simulink model "rpoco16"  (R2013a)
settings: Solver=VariableStepDiscrete  SolverMode=SingleTasking  StartTime=0.0  StopTime=10.0  RelTol=1e-3
libraries: xbsIndex_r4 x7152, casper_library_misc x156, casper_library_multipliers x68, casper_library_sources x8, xps_library x5, casper_library_delays x1
(part 2 of 84)

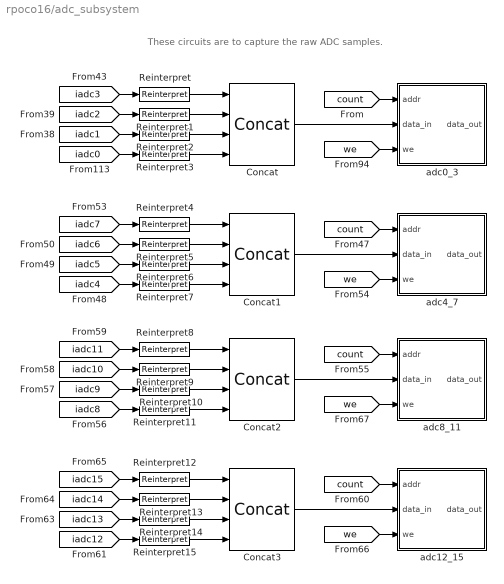
== system rpoco16/adc_subsystem ==
  note: These circuits are to capture the raw ADC samples.
  Concat{,1..3} (4 alike) : xbsIndex_r4/Concat  num_inputs=4  dbl_ovrd=off  block_type=concat
  Reinterpret{,1..15} (16 alike) : xbsIndex_r4/Reinterpret  force_arith_type=on  arith_type=Unsigned  force_bin_pt=on  bin_pt=0  block_type=reinterpret
      settings: infoedit="Changes signal type without altering the binary representation.   You can changed the signal between signed and unsigned, and relocate the binary point.<br><br>Hardware notes: In hardware this block costs nothing.<br><br>Example:  Suppose the input is 6 bits wide, signed, with 2 fractional bits, and the output is forced to unsigned with 0 fractional bits.  Then an input of -2.0 (1110.00 in binary 2's complement) becomes an output of 56 (111000 in binary)."
  adc0_3 : Subsystem  Tag=xps:bram  AncestorBlock=xps_library/Shared BRAM  mask{arith_type=Unsigned, addr_width=11, data_width=32, reg_prim_output=off, reg_core_output=off, optimization=Minimum_Area, data_bin_pt=0, init_vals=[1:2^10-1], sample_rate=1}
      mask prompts: arith_type "Output Data Type"; addr_width "Address width"; data_width "Data Width"; reg_prim_output "Register Primitive Output"; reg_core_output "Register Core Output"; data_bin_pt "Data Binary Point"; init_vals "Initial values (simulation only)"; sample_rate "Sample rate"
      mask init:
      | shared_bram_mask;
      mask TypeOptions arith_type: Unsigned | Signed  (2's comp)
      mask TypeOptions data_width: 8 | 16 | 32 | 64 | 128
      mask TypeOptions optimization: Minimum_Area | Low_Power
  adc12_15 : Subsystem  Tag=xps:bram  AncestorBlock=xps_library/Shared BRAM  mask{arith_type=Unsigned, addr_width=11, data_width=32, reg_prim_output=off, reg_core_output=off, optimization=Minimum_Area, data_bin_pt=0, init_vals=[1:2^10-1], sample_rate=1}
      mask prompts: arith_type "Output Data Type"; addr_width "Address width"; data_width "Data Width"; reg_prim_output "Register Primitive Output"; reg_core_output "Register Core Output"; data_bin_pt "Data Binary Point"; init_vals "Initial values (simulation only)"; sample_rate "Sample rate"
      mask init:
      | shared_bram_mask;
      mask TypeOptions arith_type: Unsigned | Signed  (2's comp)
      mask TypeOptions data_width: 8 | 16 | 32 | 64 | 128
      mask TypeOptions optimization: Minimum_Area | Low_Power
  adc4_7 : Subsystem  Tag=xps:bram  AncestorBlock=xps_library/Shared BRAM  mask{arith_type=Unsigned, addr_width=11, data_width=32, reg_prim_output=off, reg_core_output=off, optimization=Minimum_Area, data_bin_pt=0, init_vals=[1:2^10-1], sample_rate=1}
      mask prompts: arith_type "Output Data Type"; addr_width "Address width"; data_width "Data Width"; reg_prim_output "Register Primitive Output"; reg_core_output "Register Core Output"; data_bin_pt "Data Binary Point"; init_vals "Initial values (simulation only)"; sample_rate "Sample rate"
      mask init:
      | shared_bram_mask;
      mask TypeOptions arith_type: Unsigned | Signed  (2's comp)
      mask TypeOptions data_width: 8 | 16 | 32 | 64 | 128
      mask TypeOptions optimization: Minimum_Area | Low_Power
  adc8_11 : Subsystem  Tag=xps:bram  AncestorBlock=xps_library/Shared BRAM  mask{arith_type=Unsigned, addr_width=11, data_width=32, reg_prim_output=off, reg_core_output=off, optimization=Minimum_Area, data_bin_pt=0, init_vals=[1:2^10-1], sample_rate=1}
      mask prompts: arith_type "Output Data Type"; addr_width "Address width"; data_width "Data Width"; reg_prim_output "Register Primitive Output"; reg_core_output "Register Core Output"; data_bin_pt "Data Binary Point"; init_vals "Initial values (simulation only)"; sample_rate "Sample rate"
      mask init:
      | shared_bram_mask;
      mask TypeOptions arith_type: Unsigned | Signed  (2's comp)
      mask TypeOptions data_width: 8 | 16 | 32 | 64 | 128
      mask TypeOptions optimization: Minimum_Area | Low_Power
  wires:
  [count] -> adc4_7/1(addr)
  [we] -> adc4_7/3(we)
  Concat1/1 -> adc4_7/2(data_in)
  Reinterpret4/1 -> Concat1/1
  Reinterpret5/1 -> Concat1/2
  Reinterpret6/1 -> Concat1/3
  Reinterpret7/1 -> Concat1/4
  [iadc7] -> Reinterpret4/1
  [iadc6] -> Reinterpret5/1
  [iadc5] -> Reinterpret6/1
  [iadc4] -> Reinterpret7/1
  Reinterpret13/1 -> Concat3/2
  Reinterpret14/1 -> Concat3/3
  Reinterpret15/1 -> Concat3/4
  [iadc15] -> Reinterpret12/1
  [iadc14] -> Reinterpret13/1
  [iadc13] -> Reinterpret14/1
  [iadc12] -> Reinterpret15/1
  Reinterpret8/1 -> Concat2/1
  Reinterpret9/1 -> Concat2/2
  Reinterpret10/1 -> Concat2/3
  Reinterpret11/1 -> Concat2/4
  [iadc11] -> Reinterpret8/1
  [iadc10] -> Reinterpret9/1
  [iadc9] -> Reinterpret10/1
  [iadc8] -> Reinterpret11/1
  [count] -> adc12_15/1(addr)
  [we] -> adc12_15/3(we)
  Reinterpret12/1 -> Concat3/1
  Concat3/1 -> adc12_15/2(data_in)
  [count] -> adc8_11/1(addr)
  Concat2/1 -> adc8_11/2(data_in)
  [we] -> adc8_11/3(we)
  Reinterpret2/1 -> Concat/3
  Reinterpret1/1 -> Concat/2
  [iadc3] -> Reinterpret/1
  Reinterpret/1 -> Concat/1
  [iadc1] -> Reinterpret2/1
  Reinterpret3/1 -> Concat/4
  Concat/1 -> adc0_3/2(data_in)
  [count] -> adc0_3/1(addr)
  [we] -> adc0_3/3(we)
  [iadc0] -> Reinterpret3/1
  [iadc2] -> Reinterpret1/1

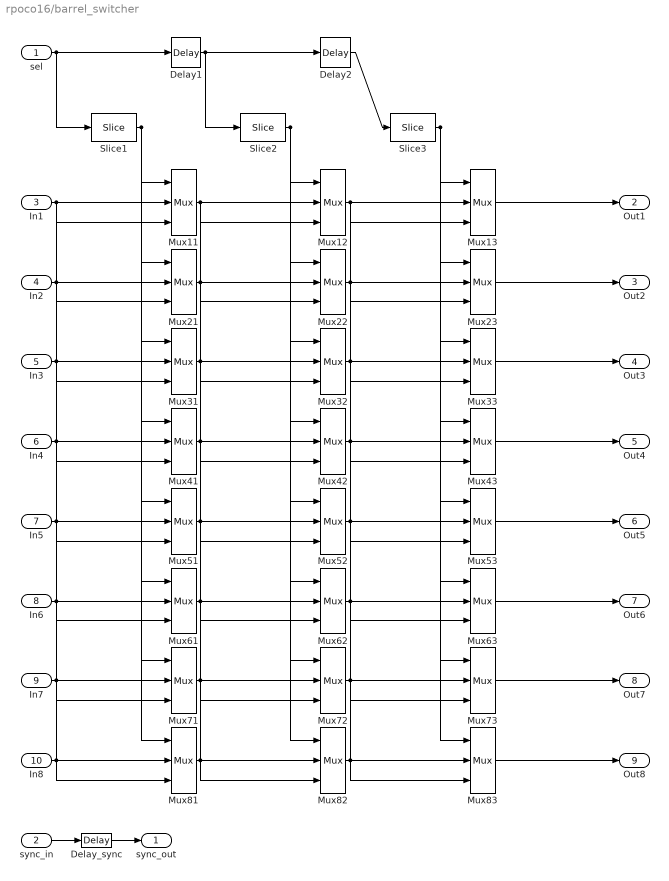
== system rpoco16/barrel_switcher ==
  sel : Inport
  sync_in : Inport  Port=2
  In1 : Inport  Port=3
  In2 : Inport  Port=4
  In3 : Inport  Port=5
  In4 : Inport  Port=6
  In5 : Inport  Port=7
  In6 : Inport  Port=8
  In7 : Inport  Port=9
  In8 : Inport  Port=10
  Delay1 : xbsIndex_r4/Delay  rst=off  infoeditControl=Selection of Reset will increase slice count due to use of real FFs and instead of SRLs  en=off  latency=1  dbl_ovrd=off  reg_retiming=on  block_type=delay
  Delay2 : xbsIndex_r4/Delay  rst=off  infoeditControl=Selection of Reset will increase slice count due to use of real FFs and instead of SRLs  en=off  latency=1  dbl_ovrd=off  reg_retiming=on  block_type=delay
  Delay_sync : xbsIndex_r4/Delay  rst=off  infoeditControl=Selection of Reset will increase slice count due to use of real FFs and instead of SRLs  en=off  latency=3  dbl_ovrd=off  reg_retiming=on  block_type=delay
  Mux{11..13,21..23,31..33,41..43,51..53,61..63,71..73,81..83} (24 alike) : xbsIndex_r4/Mux  inputs=2  en=off  latency=1  precision=Full  arith_type=Unsigned  n_bits=16  bin_pt=14  quantization=Truncate  overflow=Wrap  dbl_ovrd=off  block_type=mux
  Slice1 : xbsIndex_r4/Slice  nbits=1  boolean_output=off  mode=Upper Bit Location + Width  bit1=-0  base1=MSB of Input  bit0=0  base0=LSB of Input  dbl_ovrd=off  block_type=slice
  Slice2 : xbsIndex_r4/Slice  nbits=1  boolean_output=off  mode=Upper Bit Location + Width  bit1=-1  base1=MSB of Input  bit0=0  base0=LSB of Input  dbl_ovrd=off  block_type=slice
  Slice3 : xbsIndex_r4/Slice  nbits=1  boolean_output=off  mode=Upper Bit Location + Width  bit1=-2  base1=MSB of Input  bit0=0  base0=LSB of Input  dbl_ovrd=off  block_type=slice
  sync_out : Outport
  Out1 : Outport  Port=2
  Out2 : Outport  Port=3
  Out3 : Outport  Port=4
  Out4 : Outport  Port=5
  Out5 : Outport  Port=6
  Out6 : Outport  Port=7
  Out7 : Outport  Port=8
  Out8 : Outport  Port=9
  wires:
  sync_in/1 -> Delay_sync/1
  Delay_sync/1 -> sync_out/1
  sel/1 -> Slice1/1, Delay1/1
  Delay1/1 -> Delay2/1, Slice2/1
  Delay2/1 -> Slice3/1
  Slice1/1 -> Mux11/1, Mux21/1, Mux31/1, Mux41/1, Mux51/1, Mux61/1, Mux71/1, Mux81/1
  Slice2/1 -> Mux12/1, Mux22/1, Mux32/1, Mux42/1, Mux52/1, Mux62/1, Mux72/1, Mux82/1
  Slice3/1 -> Mux13/1, Mux23/1, Mux33/1, Mux43/1, Mux53/1, Mux63/1, Mux73/1, Mux83/1
  In1/1 -> Mux11/2, Mux51/3
  Mux13/1 -> Out1/1
  In2/1 -> Mux21/2, Mux61/3
  Mux23/1 -> Out2/1
  In3/1 -> Mux31/2, Mux71/3
  Mux33/1 -> Out3/1
  In4/1 -> Mux41/2, Mux81/3
  Mux43/1 -> Out4/1
  In5/1 -> Mux51/2, Mux11/3
  Mux53/1 -> Out5/1
  In6/1 -> Mux61/2, Mux21/3
  Mux63/1 -> Out6/1
  In7/1 -> Mux71/2, Mux31/3
  Mux73/1 -> Out7/1
  In8/1 -> Mux81/2, Mux41/3
  Mux83/1 -> Out8/1
  Mux11/1 -> Mux12/2, Mux72/3
  Mux12/1 -> Mux13/2, Mux83/3
  Mux21/1 -> Mux22/2, Mux82/3
  Mux22/1 -> Mux23/2, Mux13/3
  Mux31/1 -> Mux32/2, Mux12/3
  Mux32/1 -> Mux33/2, Mux23/3
  Mux41/1 -> Mux42/2, Mux22/3
  Mux42/1 -> Mux43/2, Mux33/3
  Mux51/1 -> Mux52/2, Mux32/3
  Mux52/1 -> Mux53/2, Mux43/3
  Mux61/1 -> Mux62/2, Mux42/3
  Mux62/1 -> Mux63/2, Mux53/3
  Mux71/1 -> Mux72/2, Mux52/3
  Mux72/1 -> Mux73/2, Mux63/3
  Mux81/1 -> Mux82/2, Mux62/3
  Mux82/1 -> Mux83/2, Mux73/3

== system rpoco16/ctrl_sw ==
  sim_1 : Inport
  io_delay : xbsIndex_r4/Delay  rst=off  infoeditControl=Selection of Reset will increase slice count due to use of real FFs and instead of SRLs  en=off  latency=0  dbl_ovrd=off  reg_retiming=on  block_type=delay
  reint1 : xbsIndex_r4/Reinterpret  force_arith_type=on  arith_type=Unsigned  force_bin_pt=on  bin_pt=0  block_type=reinterpret
  rpoco16_ctrl_sw_user_data_out : xbsIndex_r4/Gateway In  gui_display_data_type=Fixed-point  arith_type=Unsigned  n_bits=32  bin_pt=0  preci_type=Single  exp_width=8  frac_width=24  quantization="Round  (unbiased: +/- Inf)"  overflow=Saturate  period=1  dbl_ovrd=off  timing_constraint=None  locs_specified=off  LOCs={}  UseAsADC=off  ADCChannel='1'  inherit_from_input=off  hdl_port=on  block_type=gatewayin
  slice_reg : xbsIndex_r4/Slice  nbits=32  boolean_output=off  mode=Lower Bit Location + Width  bit1=0  base1=MSB of Input  bit0=0  base0=LSB of Input  dbl_ovrd=off  block_type=slice
  in_reg : Outport
  wires:
  rpoco16_ctrl_sw_user_data_out/1 -> io_delay/1
  sim_1/1 -> rpoco16_ctrl_sw_user_data_out/1
  io_delay/1 -> slice_reg/1
  slice_reg/1 -> reint1/1
  reint1/1 -> in_reg/1

== system rpoco16/delay ==
  note: Delay data is a 32 bit input, and delayi is a
      | 4 bit output. Max delay is 16 clocks.
  BitBasher : xbsIndex_r4/BitBasher  bitexpr=|  display_expr=off  sr_1=1  arith_type1=Unsigned  bin_pt1=0  sr_2=2  arith_type2=Unsigned  bin_pt2=0  sr_3=3  arith_type3=Unsigned  bin_pt3=0  sr_4=4  arith_type4=Unsigned  bin_pt4=0  dbl_ovrd=off  block_type=bitbasher
      | <html><head><meta name="qrichtext" content="1" /><style type="text/css">
      | p, li { white-space: pre-wrap; }
      | </style></head><body style=" font-family:'MS Shell Dlg 2'; font-size:8.25pt; font-weight:400; font-style:normal;">
      | <p style=" margin-top:12px; margin-bottom:12px; margin-left:0px; margin-right:0px; -qt-block-indent:0; text-indent:0px; font-family:'MS Shell Dlg'; font-size:8pt;">delay0={delay[3:0]}<br />delay1={delay[7:4]}<br />delay2={delay[11:8]}<br />delay3={delay[15:12]}</p></body></html>
      settings: block_version=10.1.3
  BitBasher1 : xbsIndex_r4/BitBasher  bitexpr=|  display_expr=off  sr_1=1  arith_type1=Unsigned  bin_pt1=0  sr_2=2  arith_type2=Unsigned  bin_pt2=0  sr_3=3  arith_type3=Unsigned  bin_pt3=0  sr_4=4  arith_type4=Unsigned  bin_pt4=0  dbl_ovrd=off  block_type=bitbasher
      | <html><head><meta name="qrichtext" content="1" /><style type="text/css">
      | p, li { white-space: pre-wrap; }
      | </style></head><body style=" font-family:'MS Shell Dlg 2'; font-size:8.25pt; font-weight:400; font-style:normal;">
      | <p style=" margin-top:12px; margin-bottom:12px; margin-left:0px; margin-right:0px; -qt-block-indent:0; text-indent:0px; font-family:'MS Shell Dlg'; font-size:8pt;">delay4={delay[19:16]}<br />delay5={delay[23:20]}<br />delay6={delay[27:24]}<br />delay7={delay[31:28]}</p></body></html>
      settings: block_version=10.1.3
  Constant : Constant
  delay_data : Subsystem  Tag=xps:sw_reg  AncestorBlock=xps_library/software register  mask(swreg){mode=one value, io_dir=From Processor, io_delay=0, sample_period=1, names=reg, bitwidths=32, arith_types=0, bin_pts=0, sim_port=on, show_format=off}
      mask prompts: io_dir "I/O direction"; io_delay "I/O delay"; sample_period "Sample period"; names "Name:"; bitwidths "Bitwidth:"; arith_types "Type (ufix=0, fix=1, bool=2):"; bin_pts "Binary pt:"; sim_port "Provide sim input/output?"; show_format "Print format string?"
      mask init:
      | swreg_init(gcb)
      settings: AttributesFormatString=1input
      mask TypeOptions mode: one value | fields of equal size | fields of arbitrary size
      mask Callback mode: swreg_cb(gcb);
      mask TypeOptions io_dir: To Processor | From Processor
      mask Callback io_dir:
      | mask_enables = get_param(gcb, 'MaskEnables');
      | mask_names = get_param(gcb, 'MaskNames');
      | if strcmp(get_param(gcb, 'io_dir'), 'To Processor'),
      |     mask_enables{ismember(mask_names, 'sample_period')} = 'off';
      | else
      |     mask_enables{ismember(mask_names, 'sample_period')} = 'on';
      | end
      | set_param(gcb, 'MaskEnables', mask_enables);
      mask Callback bitwidths: swreg_maskcheck(gcb);
      mask Callback arith_types: [numios, ~, ~, ~, current_types] = swreg_maskcheck(gcb);
      mask Callback bin_pts: swreg_maskcheck(gcb);
  tag scope: delay0=global, delay10=global, delay11=global, delay12=global, delay13=global, delay14=global, delay15=global, delay1=global, delay2=global, delay3=global, delay4=global, delay5=global, delay6=global, delay7=global, delay8=global, delay9=global
  wires:
  delay_data/1(in_reg) -> BitBasher1/1, BitBasher/1
  Constant/1 -> delay_data/1(sim_1)
  BitBasher/1 -> [delay1], [delay0]
  BitBasher/2 -> [delay3], [delay2]
  BitBasher/3 -> [delay5], [delay4]
  BitBasher/4 -> [delay7], [delay6]
  BitBasher1/1 -> [delay9], [delay8]
  BitBasher1/2 -> [delay11], [delay10]
  BitBasher1/3 -> [delay13], [delay12]
  BitBasher1/4 -> [delay15], [delay14]

== system rpoco16/edge ==
  in : Inport
  Delay : xbsIndex_r4/Delay  rst=off  infoeditControl=Selection of Reset will increase slice count due to use of real FFs and instead of SRLs  en=off  latency=1  dbl_ovrd=off  reg_retiming=off  block_type=delay
      settings: xl_area=[0, 0, 0, 0, 0, 0, 0]
  Inverter : xbsIndex_r4/Inverter  en=off  latency=0  dbl_ovrd=off  block_type=inv
      settings: xl_area=[0, 0, 0, 0, 0, 0, 0]
  edge_op : xbsIndex_r4/Logical  logical_function=XNOR  inputs=2  en=off  latency=0  precision=Full  arith_type=Unsigned  n_bits=8  bin_pt=2  align_bp=on  dbl_ovrd=off  block_type=logical
      settings: xl_area=[0, 0, 0, 0, 0, 0, 0]
  out : Outport
  wires:
  Inverter/1 -> edge_op/1
  edge_op/1 -> out/1
  in/1 -> Inverter/1, Delay/1
  Delay/1 -> edge_op/2

== system rpoco16/eq_coeff ==
  sim_1 : Inport
  io_delay : xbsIndex_r4/Delay  rst=off  infoeditControl=Selection of Reset will increase slice count due to use of real FFs and instead of SRLs  en=off  latency=0  dbl_ovrd=off  reg_retiming=on  block_type=delay
  reint1 : xbsIndex_r4/Reinterpret  force_arith_type=on  arith_type=Unsigned  force_bin_pt=on  bin_pt=0  block_type=reinterpret
  rpoco16_eq_coeff_user_data_out : xbsIndex_r4/Gateway In  gui_display_data_type=Fixed-point  arith_type=Unsigned  n_bits=32  bin_pt=0  preci_type=Single  exp_width=8  frac_width=24  quantization="Round  (unbiased: +/- Inf)"  overflow=Saturate  period=1  dbl_ovrd=off  timing_constraint=None  locs_specified=off  LOCs={}  UseAsADC=off  ADCChannel='1'  inherit_from_input=off  hdl_port=on  block_type=gatewayin
  slice_reg : xbsIndex_r4/Slice  nbits=32  boolean_output=off  mode=Lower Bit Location + Width  bit1=0  base1=MSB of Input  bit0=0  base0=LSB of Input  dbl_ovrd=off  block_type=slice
  in_reg : Outport
  wires:
  rpoco16_eq_coeff_user_data_out/1 -> io_delay/1
  sim_1/1 -> rpoco16_eq_coeff_user_data_out/1
  io_delay/1 -> slice_reg/1
  slice_reg/1 -> reint1/1
  reint1/1 -> in_reg/1

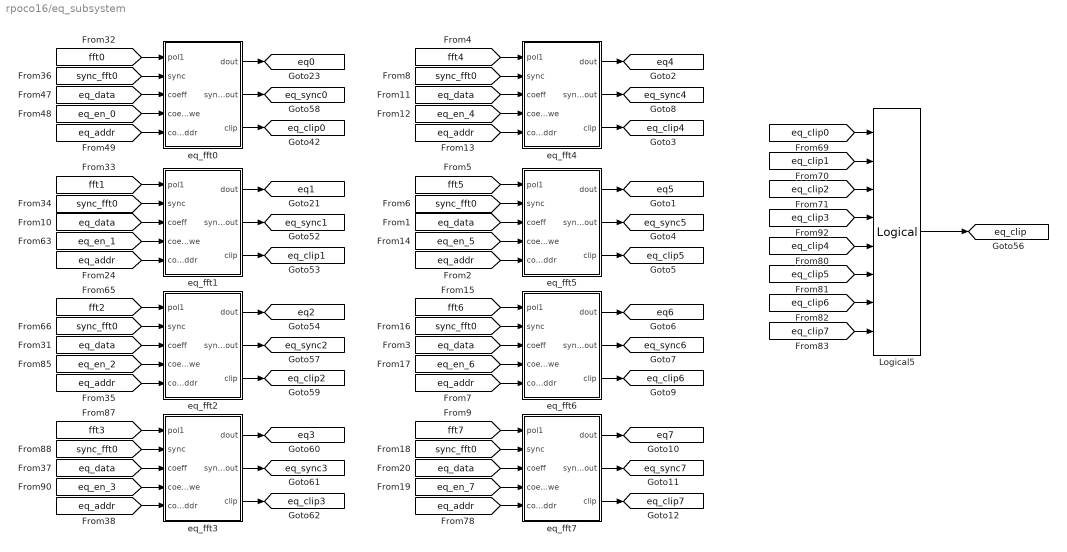
== system rpoco16/eq_subsystem ==
  Logical5 : xbsIndex_r4/Logical  logical_function=OR  inputs=8  en=off  latency=0  precision=Full  arith_type=Unsigned  n_bits=8  bin_pt=2  align_bp=on  dbl_ovrd=off  block_type=logical
      settings: xl_area=[0, 0, 0, 0, 0, 0, 0]
  eq_fft0 : Subsystem  mask{nchan=11}
      mask prompts: nchan "FFT Channels (2^?):"
  eq_fft1 : Subsystem  mask{nchan=11}
      mask prompts: nchan "FFT Channels (2^?):"
  eq_fft2 : Subsystem  mask{nchan=11}
      mask prompts: nchan "FFT Channels (2^?):"
  eq_fft3 : Subsystem  mask{nchan=11}
      mask prompts: nchan "FFT Channels (2^?):"
  eq_fft4 : Subsystem  mask{nchan=11}
      mask prompts: nchan "FFT Channels (2^?):"
  eq_fft5 : Subsystem  mask{nchan=11}
      mask prompts: nchan "FFT Channels (2^?):"
  eq_fft6 : Subsystem  mask{nchan=11}
      mask prompts: nchan "FFT Channels (2^?):"
  eq_fft7 : Subsystem  mask{nchan=11}
      mask prompts: nchan "FFT Channels (2^?):"
  tag scope: eq0=global, eq1=global, eq2=global, eq3=global, eq4=global, eq5=global, eq6=global, eq7=global, eq_clip0=global, eq_clip1=global, eq_clip2=global, eq_clip3=global, eq_clip4=global, eq_clip5=global, eq_clip6=global, eq_clip7=global, eq_clip=global, eq_sync0=global, eq_sync1=global, eq_sync2=global, eq_sync3=global, eq_sync4=global, eq_sync5=global, eq_sync6=global, eq_sync7=global
  wires:
  Logical5/1 -> [eq_clip]
  [eq_clip0] -> Logical5/1
  [eq_clip1] -> Logical5/2
  [eq_clip2] -> Logical5/3
  [eq_clip3] -> Logical5/4
  [eq_data] -> eq_fft1/3(coeff)
  eq_fft0/1(dout) -> [eq0]
  eq_fft0/2(sync_out) -> [eq_sync0]
  [fft0] -> eq_fft0/1(pol1)
  [eq_data] -> eq_fft0/3(coeff)
  [eq_en_0] -> eq_fft0/4(coeff_we)
  eq_fft0/3(clip) -> [eq_clip0]
  [sync_fft0] -> eq_fft0/2(sync)
  [eq_addr] -> eq_fft0/5(coeff_addr)
  [fft1] -> eq_fft1/1(pol1)
  [sync_fft0] -> eq_fft1/2(sync)
  [eq_en_1] -> eq_fft1/4(coeff_we)
  [eq_addr] -> eq_fft1/5(coeff_addr)
  [fft2] -> eq_fft2/1(pol1)
  [sync_fft0] -> eq_fft2/2(sync)
  [eq_data] -> eq_fft2/3(coeff)
  [eq_en_2] -> eq_fft2/4(coeff_we)
  [eq_addr] -> eq_fft2/5(coeff_addr)
  [fft3] -> eq_fft3/1(pol1)
  [sync_fft0] -> eq_fft3/2(sync)
  [eq_data] -> eq_fft3/3(coeff)
  [eq_en_3] -> eq_fft3/4(coeff_we)
  [eq_addr] -> eq_fft3/5(coeff_addr)
  eq_fft1/1(dout) -> [eq1]
  eq_fft1/2(sync_out) -> [eq_sync1]
  eq_fft1/3(clip) -> [eq_clip1]
  eq_fft2/1(dout) -> [eq2]
  eq_fft2/2(sync_out) -> [eq_sync2]
  eq_fft2/3(clip) -> [eq_clip2]
  eq_fft3/1(dout) -> [eq3]
  eq_fft3/2(sync_out) -> [eq_sync3]
  eq_fft3/3(clip) -> [eq_clip3]
  [eq_data] -> eq_fft5/3(coeff)
  eq_fft4/1(dout) -> [eq4]
  eq_fft4/2(sync_out) -> [eq_sync4]
  [fft4] -> eq_fft4/1(pol1)
  [eq_data] -> eq_fft4/3(coeff)
  [eq_en_4] -> eq_fft4/4(coeff_we)
  eq_fft4/3(clip) -> [eq_clip4]
  [sync_fft0] -> eq_fft4/2(sync)
  [eq_addr] -> eq_fft4/5(coeff_addr)
  [fft5] -> eq_fft5/1(pol1)
  [sync_fft0] -> eq_fft5/2(sync)
  [eq_en_5] -> eq_fft5/4(coeff_we)
  [eq_addr] -> eq_fft5/5(coeff_addr)
  [fft6] -> eq_fft6/1(pol1)
  [sync_fft0] -> eq_fft6/2(sync)
  [eq_data] -> eq_fft6/3(coeff)
  [eq_en_6] -> eq_fft6/4(coeff_we)
  [eq_addr] -> eq_fft6/5(coeff_addr)
  eq_fft5/1(dout) -> [eq5]
  eq_fft5/2(sync_out) -> [eq_sync5]
  eq_fft5/3(clip) -> [eq_clip5]
  eq_fft6/1(dout) -> [eq6]
  eq_fft6/2(sync_out) -> [eq_sync6]
  eq_fft6/3(clip) -> [eq_clip6]
  [fft7] -> eq_fft7/1(pol1)
  [sync_fft0] -> eq_fft7/2(sync)
  [eq_data] -> eq_fft7/3(coeff)
  [eq_en_7] -> eq_fft7/4(coeff_we)
  [eq_addr] -> eq_fft7/5(coeff_addr)
  eq_fft7/1(dout) -> [eq7]
  eq_fft7/2(sync_out) -> [eq_sync7]
  eq_fft7/3(clip) -> [eq_clip7]
  [eq_clip4] -> Logical5/5
  [eq_clip5] -> Logical5/6
  [eq_clip6] -> Logical5/7
  [eq_clip7] -> Logical5/8

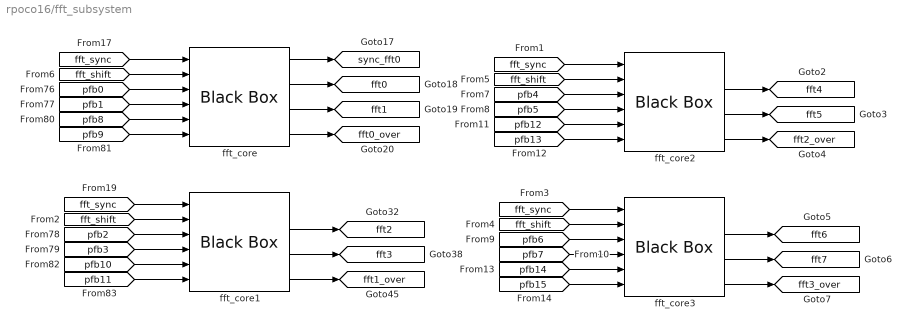
== system rpoco16/fft_subsystem ==
  fft_core{,1..3} (4 alike) : xbsIndex_r4/Black Box  init_code=fft_core_v6_config  sim_method=Inactive  verbose=off  block_type=blackbox2
  tag scope: fft0=global, fft0_over=global, fft1=global, fft1_over=global, fft2=global, fft2_over=global, fft3=global, fft3_over=global, fft4=global, fft5=global, fft6=global, fft7=global, sync_fft0=global
  wires:
  [pfb1] -> fft_core/4
  [pfb11] -> fft_core1/6
  [pfb3] -> fft_core1/4
  [pfb0] -> fft_core/3
  fft_core/4 -> [fft0_over]
  [fft_sync] -> fft_core/1
  [pfb8] -> fft_core/5
  fft_core1/3 -> [fft3]
  fft_core/2 -> [fft0]
  [pfb2] -> fft_core1/3
  [fft_sync] -> fft_core1/1
  [pfb9] -> fft_core/6
  fft_core1/4 -> [fft1_over]
  [fft_shift] -> fft_core/2
  fft_core1/2 -> [fft2]
  [fft_shift] -> fft_core1/2
  fft_core/3 -> [fft1]
  [pfb10] -> fft_core1/5
  fft_core/1 -> [sync_fft0]
  [pfb5] -> fft_core2/4
  [pfb15] -> fft_core3/6
  [pfb7] -> fft_core3/4
  [pfb4] -> fft_core2/3
  fft_core2/4 -> [fft2_over]
  [fft_sync] -> fft_core2/1
  [pfb12] -> fft_core2/5
  fft_core3/3 -> [fft7]
  fft_core2/2 -> [fft4]
  [pfb6] -> fft_core3/3
  [fft_sync] -> fft_core3/1
  [pfb13] -> fft_core2/6
  fft_core3/4 -> [fft3_over]
  [fft_shift] -> fft_core2/2
  fft_core3/2 -> [fft6]
  [fft_shift] -> fft_core3/2
  fft_core2/3 -> [fft5]
  [pfb14] -> fft_core3/5

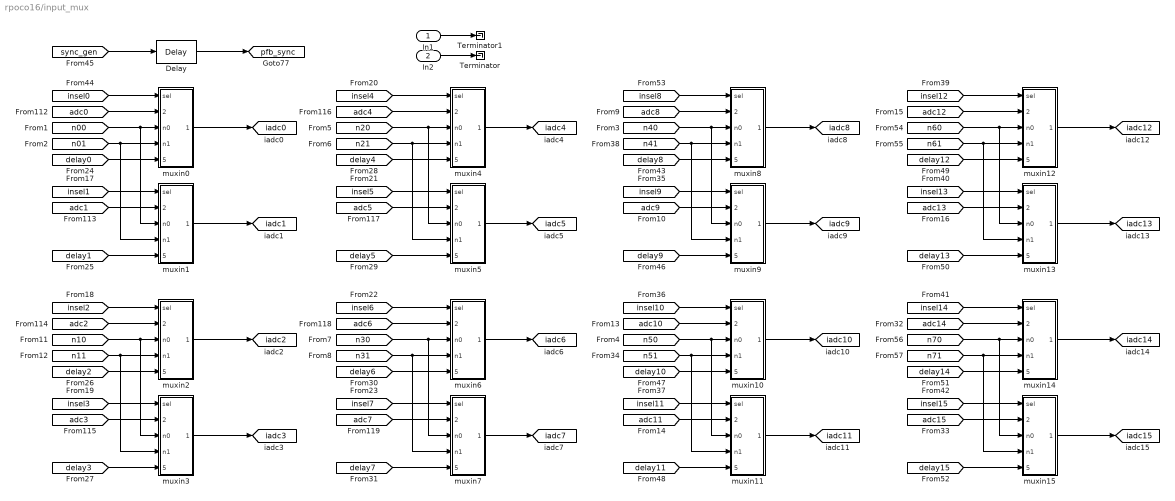
== system rpoco16/input_mux ==
  In1 : Inport
  In2 : Inport  Port=2
  Delay : xbsIndex_r4/Delay  rst=off  infoeditControl=Selection of Reset will increase slice count due to use of real FFs and instead of SRLs  en=off  latency=2  dbl_ovrd=off  reg_retiming=off  block_type=delay
  Terminator : Terminator
  Terminator1 : Terminator
  muxin0 : Subsystem
  muxin1 : Subsystem
  muxin10 : Subsystem
  muxin11 : Subsystem
  muxin12 : Subsystem
  muxin13 : Subsystem
  muxin14 : Subsystem
  muxin15 : Subsystem
  muxin2 : Subsystem
  muxin3 : Subsystem
  muxin4 : Subsystem
  muxin5 : Subsystem
  muxin6 : Subsystem
  muxin7 : Subsystem
  muxin8 : Subsystem
  muxin9 : Subsystem
  tag scope: iadc0=global, iadc10=global, iadc11=global, iadc12=global, iadc13=global, iadc14=global, iadc15=global, iadc1=global, iadc2=global, iadc3=global, iadc4=global, iadc5=global, iadc6=global, iadc7=global, iadc8=global, iadc9=global, pfb_sync=global
  wires:
  [insel0] -> muxin0/1(sel)
  [adc0] -> muxin0/2(adc)
  [n00] -> muxin0/3(n0), muxin1/3(n0)
  [n01] -> muxin0/4(n1), muxin1/4(n1)
  [delay0] -> muxin0/5(delay)
  [insel1] -> muxin1/1(sel)
  [adc1] -> muxin1/2(adc)
  [delay1] -> muxin1/5(delay)
  [insel2] -> muxin2/1(sel)
  [adc2] -> muxin2/2(adc)
  [n10] -> muxin3/3(n0), muxin2/3(n0)
  [n11] -> muxin3/4(n1), muxin2/4(n1)
  [delay2] -> muxin2/5(delay)
  [insel3] -> muxin3/1(sel)
  [adc3] -> muxin3/2(adc)
  [delay3] -> muxin3/5(delay)
  [insel4] -> muxin4/1(sel)
  [adc4] -> muxin4/2(adc)
  [n20] -> muxin5/3(n0), muxin4/3(n0)
  [n21] -> muxin5/4(n1), muxin4/4(n1)
  [delay4] -> muxin4/5(delay)
  [insel5] -> muxin5/1(sel)
  [adc5] -> muxin5/2(adc)
  [delay5] -> muxin5/5(delay)
  [insel6] -> muxin6/1(sel)
  [adc6] -> muxin6/2(adc)
  [n30] -> muxin7/3(n0), muxin6/3(n0)
  [n31] -> muxin7/4(n1), muxin6/4(n1)
  [delay6] -> muxin6/5(delay)
  [insel7] -> muxin7/1(sel)
  [adc7] -> muxin7/2(adc)
  [delay7] -> muxin7/5(delay)
  [sync_gen] -> Delay/1
  Delay/1 -> [pfb_sync]
  In1/1 -> Terminator1/1
  In2/1 -> Terminator/1
  [insel8] -> muxin8/1(sel)
  [adc8] -> muxin8/2(adc)
  [n40] -> muxin9/3(n0), muxin8/3(n0)
  [n41] -> muxin9/4(n1), muxin8/4(n1)
  [delay8] -> muxin8/5(delay)
  [insel9] -> muxin9/1(sel)
  [adc9] -> muxin9/2(adc)
  [delay9] -> muxin9/5(delay)
  [insel10] -> muxin10/1(sel)
  [adc10] -> muxin10/2(adc)
  [n50] -> muxin10/3(n0), muxin11/3(n0)
  [n51] -> muxin10/4(n1), muxin11/4(n1)
  [delay10] -> muxin10/5(delay)
  [insel11] -> muxin11/1(sel)
  [adc11] -> muxin11/2(adc)
  [delay11] -> muxin11/5(delay)
  [insel12] -> muxin12/1(sel)
  [adc12] -> muxin12/2(adc)
  [n60] -> muxin12/3(n0), muxin13/3(n0)
  [n61] -> muxin12/4(n1), muxin13/4(n1)
  [delay12] -> muxin12/5(delay)
  [insel13] -> muxin13/1(sel)
  [adc13] -> muxin13/2(adc)
  [delay13] -> muxin13/5(delay)
  [insel14] -> muxin14/1(sel)
  [adc14] -> muxin14/2(adc)
  [n70] -> muxin14/3(n0), muxin15/3(n0)
  [n71] -> muxin14/4(n1), muxin15/4(n1)
  [delay14] -> muxin14/5(delay)
  [insel15] -> muxin15/1(sel)
  [adc15] -> muxin15/2(adc)
  [delay15] -> muxin15/5(delay)
  muxin0/1(out) -> [iadc0]
  muxin1/1(out) -> [iadc1]
  muxin2/1(out) -> [iadc2]
  muxin3/1(out) -> [iadc3]
  muxin4/1(out) -> [iadc4]
  muxin5/1(out) -> [iadc5]
  muxin6/1(out) -> [iadc6]
  muxin7/1(out) -> [iadc7]
  muxin8/1(out) -> [iadc8]
  muxin9/1(out) -> [iadc9]
  muxin10/1(out) -> [iadc10]
  muxin11/1(out) -> [iadc11]
  muxin12/1(out) -> [iadc12]
  muxin13/1(out) -> [iadc13]
  muxin14/1(out) -> [iadc14]
  muxin15/1(out) -> [iadc15]

== system rpoco16/insel ==
  note: insel is a 32 bit input. every 4 bits represents a
      | selection input in the mux subsystem block. The inputs
      | are as follows:0=adc, 1=noise0, 2=noise1, 3=constant (0)
  BitBasher : xbsIndex_r4/BitBasher  bitexpr=|  display_expr=off  sr_1=1  arith_type1=Unsigned  bin_pt1=0  sr_2=2  arith_type2=Unsigned  bin_pt2=0  sr_3=3  arith_type3=Unsigned  bin_pt3=0  sr_4=4  arith_type4=Unsigned  bin_pt4=0  dbl_ovrd=off  block_type=bitbasher
      | <!DOCTYPE HTML PUBLIC "-//W3C//DTD HTML 4.0//EN" "http://www.w3.org/TR/REC-html40/strict.dtd">
      | <html><head><meta name="qrichtext" content="1" /><style type="text/css">
      | p, li { white-space: pre-wrap; }
      | </style></head><body style=" font-family:'Sans Serif'; font-size:12pt; font-weight:400; font-style:normal;">
      | <p style=" margin-top:12px; margin-bottom:12px; margin-left:0px; margin-right:0px; -qt-block-indent:0; text-indent:0px;"><span style=" font-family:'MS Shell Dlg'; font-size:8pt;">insel0={insel[1:0]}<br />insel1={insel[3:2]}<br />insel2={insel[5:4]}<br />insel3={insel[7:6]}</span></p></body></html>
      settings: block_version=10.1.3
  BitBasher1 : xbsIndex_r4/BitBasher  bitexpr=|  display_expr=off  sr_1=1  arith_type1=Unsigned  bin_pt1=0  sr_2=2  arith_type2=Unsigned  bin_pt2=0  sr_3=3  arith_type3=Unsigned  bin_pt3=0  sr_4=4  arith_type4=Unsigned  bin_pt4=0  dbl_ovrd=off  block_type=bitbasher
      | <!DOCTYPE HTML PUBLIC "-//W3C//DTD HTML 4.0//EN" "http://www.w3.org/TR/REC-html40/strict.dtd">
      | <html><head><meta name="qrichtext" content="1" /><style type="text/css">
      | p, li { white-space: pre-wrap; }
      | </style></head><body style=" font-family:'Sans Serif'; font-size:12pt; font-weight:400; font-style:normal;">
      | <p style=" margin-top:12px; margin-bottom:12px; margin-left:0px; margin-right:0px; -qt-block-indent:0; text-indent:0px;"><span style=" font-family:'MS Shell Dlg'; font-size:8pt;">insel0={insel[9:8]}<br />insel1={insel[11:10]}<br />insel2={insel[13:12]}<br />insel3={insel[15:14]}</span></p></body></html>
      settings: block_version=10.1.3
  BitBasher2 : xbsIndex_r4/BitBasher  bitexpr=|  display_expr=off  sr_1=1  arith_type1=Unsigned  bin_pt1=0  sr_2=2  arith_type2=Unsigned  bin_pt2=0  sr_3=3  arith_type3=Unsigned  bin_pt3=0  sr_4=4  arith_type4=Unsigned  bin_pt4=0  dbl_ovrd=off  block_type=bitbasher
      | <!DOCTYPE HTML PUBLIC "-//W3C//DTD HTML 4.0//EN" "http://www.w3.org/TR/REC-html40/strict.dtd">
      | <html><head><meta name="qrichtext" content="1" /><style type="text/css">
      | p, li { white-space: pre-wrap; }
      | </style></head><body style=" font-family:'Sans Serif'; font-size:12pt; font-weight:400; font-style:normal;">
      | <p style=" margin-top:12px; margin-bottom:12px; margin-left:0px; margin-right:0px; -qt-block-indent:0; text-indent:0px;"><span style=" font-family:'MS Shell Dlg'; font-size:8pt;">insel0={insel[17:16]}<br />insel1={insel[19:18]}<br />insel2={insel[21:20]}<br />insel3={insel[23:22]}</span></p></body></html>
      settings: block_version=10.1.3
  BitBasher3 : xbsIndex_r4/BitBasher  bitexpr=|  display_expr=off  sr_1=1  arith_type1=Unsigned  bin_pt1=0  sr_2=2  arith_type2=Unsigned  bin_pt2=0  sr_3=3  arith_type3=Unsigned  bin_pt3=0  sr_4=4  arith_type4=Unsigned  bin_pt4=0  dbl_ovrd=off  block_type=bitbasher
      | <!DOCTYPE HTML PUBLIC "-//W3C//DTD HTML 4.0//EN" "http://www.w3.org/TR/REC-html40/strict.dtd">
      | <html><head><meta name="qrichtext" content="1" /><style type="text/css">
      | p, li { white-space: pre-wrap; }
      | </style></head><body style=" font-family:'Sans Serif'; font-size:12pt; font-weight:400; font-style:normal;">
      | <p style=" margin-top:12px; margin-bottom:12px; margin-left:0px; margin-right:0px; -qt-block-indent:0; text-indent:0px;"><span style=" font-family:'MS Shell Dlg'; font-size:8pt;">insel0={insel[25:24]}<br />insel1={insel[27:26]}<br />insel2={insel[29:28]}<br />insel3={insel[31:30]}</span></p></body></html>
      settings: block_version=10.1.3
  Constant : Constant  Value=858862385
  insel_data : Subsystem  Tag=xps:sw_reg  AncestorBlock=xps_library/software register  mask(swreg){mode=one value, io_dir=From Processor, io_delay=0, sample_period=1, names=reg, bitwidths=32, arith_types=0, bin_pts=0, sim_port=on, show_format=off}
      mask prompts: io_dir "I/O direction"; io_delay "I/O delay"; sample_period "Sample period"; names "Name:"; bitwidths "Bitwidth:"; arith_types "Type (ufix=0, fix=1, bool=2):"; bin_pts "Binary pt:"; sim_port "Provide sim input/output?"; show_format "Print format string?"
      mask init:
      | swreg_init(gcb)
      settings: AttributesFormatString=1input
      mask TypeOptions mode: one value | fields of equal size | fields of arbitrary size
      mask Callback mode: swreg_cb(gcb);
      mask TypeOptions io_dir: To Processor | From Processor
      mask Callback io_dir:
      | mask_enables = get_param(gcb, 'MaskEnables');
      | mask_names = get_param(gcb, 'MaskNames');
      | if strcmp(get_param(gcb, 'io_dir'), 'To Processor'),
      |     mask_enables{ismember(mask_names, 'sample_period')} = 'off';
      | else
      |     mask_enables{ismember(mask_names, 'sample_period')} = 'on';
      | end
      | set_param(gcb, 'MaskEnables', mask_enables);
      mask Callback bitwidths: swreg_maskcheck(gcb);
      mask Callback arith_types: [numios, ~, ~, ~, current_types] = swreg_maskcheck(gcb);
      mask Callback bin_pts: swreg_maskcheck(gcb);
  tag scope: insel0=global, insel10=global, insel11=global, insel12=global, insel13=global, insel14=global, insel15=global, insel1=global, insel2=global, insel3=global, insel4=global, insel5=global, insel6=global, insel7=global, insel8=global, insel9=global
  wires:
  insel_data/1(in_reg) -> BitBasher1/1, BitBasher/1, BitBasher3/1, BitBasher2/1
  Constant/1 -> insel_data/1(sim_1)
  BitBasher/1 -> [insel0]
  BitBasher/2 -> [insel1]
  BitBasher/3 -> [insel2]
  BitBasher/4 -> [insel3]
  BitBasher1/1 -> [insel4]
  BitBasher1/4 -> [insel7]
  BitBasher1/3 -> [insel6]
  BitBasher1/2 -> [insel5]
  BitBasher2/4 -> [insel11]
  BitBasher2/3 -> [insel10]
  BitBasher2/2 -> [insel9]
  BitBasher2/1 -> [insel8]
  BitBasher3/4 -> [insel15]
  BitBasher3/3 -> [insel14]
  BitBasher3/2 -> [insel13]
  BitBasher3/1 -> [insel12]

== system rpoco16/new_raw_capture ==
  sim_1 : Inport
  io_delay : xbsIndex_r4/Delay  rst=off  infoeditControl=Selection of Reset will increase slice count due to use of real FFs and instead of SRLs  en=off  latency=0  dbl_ovrd=off  reg_retiming=on  block_type=delay
  reint1 : xbsIndex_r4/Reinterpret  force_arith_type=on  arith_type=Unsigned  force_bin_pt=on  bin_pt=0  block_type=reinterpret
  rpoco16_new_raw_capture_user_data_out : xbsIndex_r4/Gateway In  gui_display_data_type=Fixed-point  arith_type=Unsigned  n_bits=32  bin_pt=0  preci_type=Single  exp_width=8  frac_width=24  quantization="Round  (unbiased: +/- Inf)"  overflow=Saturate  period=1  dbl_ovrd=off  timing_constraint=None  locs_specified=off  LOCs={}  UseAsADC=off  ADCChannel='1'  inherit_from_input=off  hdl_port=on  block_type=gatewayin
  slice_reg : xbsIndex_r4/Slice  nbits=32  boolean_output=off  mode=Lower Bit Location + Width  bit1=0  base1=MSB of Input  bit0=0  base0=LSB of Input  dbl_ovrd=off  block_type=slice
  in_reg : Outport
  wires:
  rpoco16_new_raw_capture_user_data_out/1 -> io_delay/1
  sim_1/1 -> rpoco16_new_raw_capture_user_data_out/1
  io_delay/1 -> slice_reg/1
  slice_reg/1 -> reint1/1
  reint1/1 -> in_reg/1

== system rpoco16/new_raw_capture_trig ==
  sim_1 : Inport
  io_delay : xbsIndex_r4/Delay  rst=off  infoeditControl=Selection of Reset will increase slice count due to use of real FFs and instead of SRLs  en=off  latency=0  dbl_ovrd=off  reg_retiming=on  block_type=delay
  reint1 : xbsIndex_r4/Reinterpret  force_arith_type=on  arith_type=Unsigned  force_bin_pt=on  bin_pt=0  block_type=reinterpret
  rpoco16_new_raw_capture_trig_user_data_out : xbsIndex_r4/Gateway In  gui_display_data_type=Fixed-point  arith_type=Unsigned  n_bits=32  bin_pt=0  preci_type=Single  exp_width=8  frac_width=24  quantization="Round  (unbiased: +/- Inf)"  overflow=Saturate  period=1  dbl_ovrd=off  timing_constraint=None  locs_specified=off  LOCs={}  UseAsADC=off  ADCChannel='1'  inherit_from_input=off  hdl_port=on  block_type=gatewayin
  slice_reg : xbsIndex_r4/Slice  nbits=32  boolean_output=off  mode=Lower Bit Location + Width  bit1=0  base1=MSB of Input  bit0=0  base0=LSB of Input  dbl_ovrd=off  block_type=slice
  in_reg : Outport
  wires:
  rpoco16_new_raw_capture_trig_user_data_out/1 -> io_delay/1
  sim_1/1 -> rpoco16_new_raw_capture_trig_user_data_out/1
  io_delay/1 -> slice_reg/1
  slice_reg/1 -> reint1/1
  reint1/1 -> in_reg/1

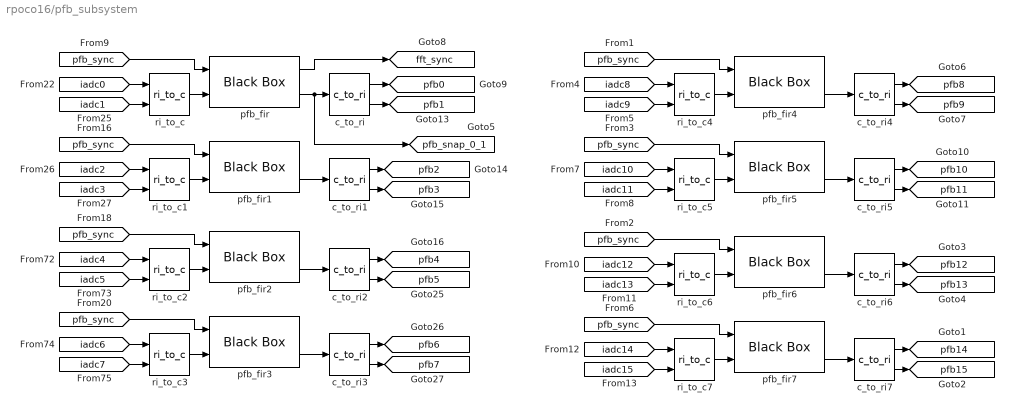
== system rpoco16/pfb_subsystem ==
  c_to_ri{,1..7} (8 alike) : casper_library_misc/c_to_ri  n_bits=18  bin_pt=17
  pfb_fir{,1..7} (8 alike) : xbsIndex_r4/Black Box  init_code=pfb_core_v6_config  sim_method=Inactive  verbose=off  block_type=blackbox2
  ri_to_c{,1..7} (8 alike) : casper_library_misc/ri_to_c
  tag scope: fft_sync=global, pfb0=global, pfb10=global, pfb11=global, pfb12=global, pfb13=global, pfb14=global, pfb15=global, pfb1=global, pfb2=global, pfb3=global, pfb4=global, pfb5=global, pfb6=global, pfb7=global, pfb8=global, pfb9=global, pfb_snap_0_1=global
  wires:
  [iadc0] -> ri_to_c/1
  ri_to_c3/1 -> pfb_fir3/2
  pfb_fir/1 -> [fft_sync]
  [iadc1] -> ri_to_c/2
  [iadc2] -> ri_to_c1/1
  [pfb_sync] -> pfb_fir2/1
  c_to_ri5/2 -> [pfb11]
  [iadc6] -> ri_to_c3/1
  c_to_ri2/2 -> [pfb5]
  [iadc10] -> ri_to_c5/1
  [pfb_sync] -> pfb_fir4/1
  ri_to_c2/1 -> pfb_fir2/2
  [iadc11] -> ri_to_c5/2
  c_to_ri4/1 -> [pfb8]
  [iadc8] -> ri_to_c4/1
  c_to_ri/1 -> [pfb0]
  c_to_ri3/2 -> [pfb7]
  [pfb_sync] -> pfb_fir3/1
  [iadc7] -> ri_to_c3/2
  c_to_ri3/1 -> [pfb6]
  pfb_fir3/2 -> c_to_ri3/1
  [iadc5] -> ri_to_c2/2
  ri_to_c5/1 -> pfb_fir5/2
  c_to_ri5/1 -> [pfb10]
  [pfb_sync] -> pfb_fir/1
  [iadc4] -> ri_to_c2/1
  pfb_fir4/2 -> c_to_ri4/1
  [pfb_sync] -> pfb_fir5/1
  c_to_ri/2 -> [pfb1]
  [iadc3] -> ri_to_c1/2
  pfb_fir2/2 -> c_to_ri2/1
  pfb_fir5/2 -> c_to_ri5/1
  pfb_fir/2 -> c_to_ri/1, [pfb_snap_0_1]
  [iadc9] -> ri_to_c4/2
  c_to_ri1/2 -> [pfb3]
  [pfb_sync] -> pfb_fir1/1
  ri_to_c4/1 -> pfb_fir4/2
  c_to_ri1/1 -> [pfb2]
  c_to_ri4/2 -> [pfb9]
  ri_to_c/1 -> pfb_fir/2
  ri_to_c1/1 -> pfb_fir1/2
  pfb_fir1/2 -> c_to_ri1/1
  c_to_ri2/1 -> [pfb4]
  c_to_ri7/2 -> [pfb15]
  [iadc14] -> ri_to_c7/1
  [pfb_sync] -> pfb_fir6/1
  [iadc15] -> ri_to_c7/2
  c_to_ri6/1 -> [pfb12]
  [iadc12] -> ri_to_c6/1
  ri_to_c7/1 -> pfb_fir7/2
  c_to_ri7/1 -> [pfb14]
  pfb_fir6/2 -> c_to_ri6/1
  [pfb_sync] -> pfb_fir7/1
  pfb_fir7/2 -> c_to_ri7/1
  [iadc13] -> ri_to_c6/2
  ri_to_c6/1 -> pfb_fir6/2
  c_to_ri6/2 -> [pfb13]

== system rpoco16/ping ==
  out_reg : Inport
  assert_reg : xbsIndex_r4/Assert  assert_type=on  type_source=Explicitly  gui_display_data_type=Fixed-point  arith_type=Unsigned  n_bits=32  bin_pt=0  preci_type=Single  exp_width=8  frac_width=24  assert_rate=off  rate_source=Explicitly  period=1  output_port=on  block_type=assert
  cast_gw : xbsIndex_r4/Convert  gui_display_data_type=Fixed-point  arith_type=Unsigned  n_bits=32  bin_pt=0  float_type=Single  exp_bits=8  fraction_bits=24  quantization=Truncate  overflow=Wrap  en=off  latency=0  dbl_ovrd=off  pipeline=off  block_type=convert
  io_delay : xbsIndex_r4/Delay  rst=off  infoeditControl=Selection of Reset will increase slice count due to use of real FFs and instead of SRLs  en=off  latency=0  dbl_ovrd=off  reg_retiming=on  block_type=delay
  reint1 : xbsIndex_r4/Reinterpret  force_arith_type=on  arith_type=Unsigned  force_bin_pt=on  bin_pt=0  block_type=reinterpret
  rpoco16_ping_user_data_in : xbsIndex_r4/Gateway Out  inherit_from_input=off  hdl_port=on  timing_constraint=None  locs_specified=off  LOCs={}  UseAsDAC=off  DACChannel='1'  block_type=gatewayout
  sim_out : Terminator
  wires:
  io_delay/1 -> cast_gw/1
  cast_gw/1 -> rpoco16_ping_user_data_in/1
  rpoco16_ping_user_data_in/1 -> sim_out/1
  out_reg/1 -> assert_reg/1
  assert_reg/1 -> reint1/1
  reint1/1 -> io_delay/1

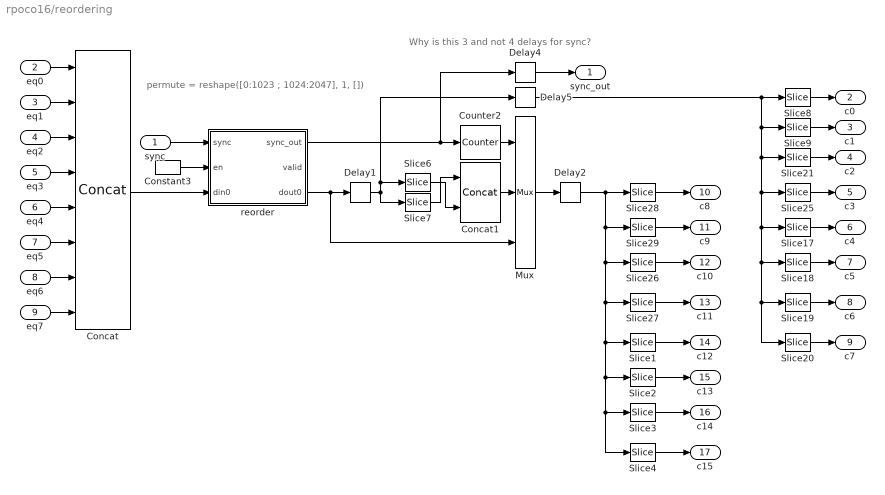
== system rpoco16/reordering ==
  note: permute = reshape([0:1023 ; 1024:2047], 1, [])
  note: Why is this 3 and not 4 delays for sync?
  sync : Inport
  eq0 : Inport  Port=2
  eq1 : Inport  Port=3
  eq2 : Inport  Port=4
  eq3 : Inport  Port=5
  eq4 : Inport  Port=6
  eq5 : Inport  Port=7
  eq6 : Inport  Port=8
  eq7 : Inport  Port=9
  Concat : xbsIndex_r4/Concat  num_inputs=8  dbl_ovrd=off  block_type=concat
      settings: block_version=10.1.3
  Concat1 : xbsIndex_r4/Concat  num_inputs=2  dbl_ovrd=off  block_type=concat
      settings: block_version=10.1.3
  Constant3 : xbsIndex_r4/Constant  const=1  gui_display_data_type=Fixed-point  arith_type=Boolean  n_bits=16  bin_pt=14  preci_type=Single  exp_width=8  frac_width=24  explicit_period=on  period=1  equ=P=C  opselect=C  inp2=PCIN>>17  opr=+  inp1=P  carry=CIN  dbl_ovrd=off  block_type=constant
  Counter2 : xbsIndex_r4/Counter  cnt_type=Free Running  cnt_to=Inf  operation=Up  start_count=0  cnt_by_val=1  arith_type=Unsigned  n_bits=1  bin_pt=0  load_pin=off  rst=on  en=off  explicit_period=on  period=1  dbl_ovrd=off  use_behavioral_HDL=off  implementation=Fabric  use_rpm=on  block_type=counter
      settings: xl_area=[0, 0, 0, 0, 0, 0, 0]
  Delay1 : xbsIndex_r4/Delay  rst=off  infoeditControl=Selection of Reset will increase slice count due to use of real FFs and instead of SRLs  en=off  latency=2  dbl_ovrd=off  reg_retiming=on  block_type=delay
      settings: xl_area=[0, 0, 0, 0, 0, 0, 0]
  Delay2 : xbsIndex_r4/Delay  rst=off  infoeditControl=Selection of Reset will increase slice count due to use of real FFs and instead of SRLs  en=off  latency=1  dbl_ovrd=off  reg_retiming=on  block_type=delay
      settings: xl_area=[0, 0, 0, 0, 0, 0, 0]
  Delay4 : xbsIndex_r4/Delay  rst=off  infoeditControl=Selection of Reset will increase slice count due to use of real FFs and instead of SRLs  en=off  latency=4  dbl_ovrd=off  reg_retiming=on  block_type=delay
      settings: xl_area=[0, 0, 0, 0, 0, 0, 0]
  Delay5 : xbsIndex_r4/Delay  rst=off  infoeditControl=Selection of Reset will increase slice count due to use of real FFs and instead of SRLs  en=off  latency=2  dbl_ovrd=off  reg_retiming=on  block_type=delay
      settings: xl_area=[0, 0, 0, 0, 0, 0, 0]
  Mux : xbsIndex_r4/Mux  inputs=2  en=off  latency=2  precision=Full  arith_type=Unsigned  n_bits=16  bin_pt=14  quantization=Truncate  overflow=Wrap  dbl_ovrd=off  block_type=mux
  Slice1 : xbsIndex_r4/Slice  nbits=2*n_bits  boolean_output=off  mode=Upper Bit Location + Width  bit1=-8*n_bits  base1=MSB of Input  bit0=16  base0=LSB of Input  dbl_ovrd=off  block_type=slice
      settings: block_version=10.1.3
  Slice17 : xbsIndex_r4/Slice  nbits=2*n_bits  boolean_output=off  mode=Upper Bit Location + Width  bit1=-8*n_bits  base1=MSB of Input  bit0=16  base0=LSB of Input  dbl_ovrd=off  block_type=slice
      settings: block_version=10.1.3
  Slice18 : xbsIndex_r4/Slice  nbits=2*n_bits  boolean_output=off  mode=Upper Bit Location + Width  bit1=-10*n_bits  base1=MSB of Input  bit0=16  base0=LSB of Input  dbl_ovrd=off  block_type=slice
      settings: block_version=10.1.3
  Slice19 : xbsIndex_r4/Slice  nbits=2*n_bits  boolean_output=off  mode=Upper Bit Location + Width  bit1=-12*n_bits  base1=MSB of Input  bit0=16  base0=LSB of Input  dbl_ovrd=off  block_type=slice
      settings: block_version=10.1.3
  Slice2 : xbsIndex_r4/Slice  nbits=2*n_bits  boolean_output=off  mode=Upper Bit Location + Width  bit1=-10*n_bits  base1=MSB of Input  bit0=16  base0=LSB of Input  dbl_ovrd=off  block_type=slice
      settings: block_version=10.1.3
  Slice20 : xbsIndex_r4/Slice  nbits=2*n_bits  boolean_output=off  mode=Upper Bit Location + Width  bit1=-14*n_bits  base1=MSB of Input  bit0=16  base0=LSB of Input  dbl_ovrd=off  block_type=slice
      settings: block_version=10.1.3
  Slice21 : xbsIndex_r4/Slice  nbits=2*n_bits  boolean_output=off  mode=Upper Bit Location + Width  bit1=-4*n_bits  base1=MSB of Input  bit0=16  base0=LSB of Input  dbl_ovrd=off  block_type=slice
      settings: block_version=10.1.3
  Slice25 : xbsIndex_r4/Slice  nbits=2*n_bits  boolean_output=off  mode=Upper Bit Location + Width  bit1=-6*n_bits  base1=MSB of Input  bit0=16  base0=LSB of Input  dbl_ovrd=off  block_type=slice
      settings: block_version=10.1.3
  Slice26 : xbsIndex_r4/Slice  nbits=2*n_bits  boolean_output=off  mode=Upper Bit Location + Width  bit1=-4*n_bits  base1=MSB of Input  bit0=16  base0=LSB of Input  dbl_ovrd=off  block_type=slice
      settings: block_version=10.1.3
  Slice27 : xbsIndex_r4/Slice  nbits=2*n_bits  boolean_output=off  mode=Upper Bit Location + Width  bit1=-6*n_bits  base1=MSB of Input  bit0=16  base0=LSB of Input  dbl_ovrd=off  block_type=slice
      settings: block_version=10.1.3
  Slice28 : xbsIndex_r4/Slice  nbits=2*n_bits  boolean_output=off  mode=Upper Bit Location + Width  bit1=0  base1=MSB of Input  bit0=16  base0=LSB of Input  dbl_ovrd=off  block_type=slice
      settings: block_version=10.1.3
  Slice29 : xbsIndex_r4/Slice  nbits=2*n_bits  boolean_output=off  mode=Upper Bit Location + Width  bit1=-2*n_bits  base1=MSB of Input  bit0=16  base0=LSB of Input  dbl_ovrd=off  block_type=slice
      settings: block_version=10.1.3
  Slice3 : xbsIndex_r4/Slice  nbits=2*n_bits  boolean_output=off  mode=Upper Bit Location + Width  bit1=-12*n_bits  base1=MSB of Input  bit0=16  base0=LSB of Input  dbl_ovrd=off  block_type=slice
      settings: block_version=10.1.3
  Slice4 : xbsIndex_r4/Slice  nbits=2*n_bits  boolean_output=off  mode=Upper Bit Location + Width  bit1=-14*n_bits  base1=MSB of Input  bit0=16  base0=LSB of Input  dbl_ovrd=off  block_type=slice
      settings: block_version=10.1.3
  Slice6 : xbsIndex_r4/Slice  nbits=4*n_bits  boolean_output=off  mode=Upper Bit Location + Width  bit1=0  base1=MSB of Input  bit0=16  base0=LSB of Input  dbl_ovrd=off  block_type=slice
      settings: block_version=10.1.3
  Slice7 : xbsIndex_r4/Slice  nbits=4*n_bits  boolean_output=off  mode=Upper Bit Location + Width  bit1=-4*n_bits  base1=MSB of Input  bit0=16  base0=LSB of Input  dbl_ovrd=off  block_type=slice
      settings: block_version=10.1.3
  Slice8 : xbsIndex_r4/Slice  nbits=2*n_bits  boolean_output=off  mode=Upper Bit Location + Width  bit1=0  base1=MSB of Input  bit0=16  base0=LSB of Input  dbl_ovrd=off  block_type=slice
      settings: block_version=10.1.3
  Slice9 : xbsIndex_r4/Slice  nbits=2*n_bits  boolean_output=off  mode=Upper Bit Location + Width  bit1=-2*n_bits  base1=MSB of Input  bit0=16  base0=LSB of Input  dbl_ovrd=off  block_type=slice
      settings: block_version=10.1.3
  reorder : Subsystem  AncestorBlock=casper_library_reorder/reorder  mask(reorder){map=getfield( getfield( get_param( gcb,'UserData' ), 'parameters'),'map'), n_bits=0, n_inputs=1, bram_latency=3, map_latency=0, fanout_latency=0, double_buffer=0, bram_map=off}
      mask prompts: map "Output Order:"; n_bits "Data width in"; n_inputs "Number of inputs"; bram_latency "BRAM Latency"; map_latency "Map Latency"; fanout_latency "Fanout latency"; double_buffer "Double Buffer"; bram_map "Use BlockRAM for Map"
      mask init:
      | reorder_init(gcb, ...
      |     'map', map, ...
      |     'n_bits', n_bits, ...
      |     'n_inputs', n_inputs, ...
      |     'bram_latency', bram_latency, ...
      |     'map_latency', map_latency, ...
      |     'fanout_latency', fanout_latency, ...
      |     'double_buffer', double_buffer, ...
      |     'bram_map', bram_map);
      settings: AttributesFormatString=order=11
      mask Help: eval('xlWeb(''http://casper.berkeley.edu/wiki/Reorder'')')
  sync_out : Outport
  c0 : Outport  Port=2
  c1 : Outport  Port=3
  c2 : Outport  Port=4
  c3 : Outport  Port=5
  c4 : Outport  Port=6
  c5 : Outport  Port=7
  c6 : Outport  Port=8
  c7 : Outport  Port=9
  c8 : Outport  Port=10
  c9 : Outport  Port=11
  c10 : Outport  Port=12
  c11 : Outport  Port=13
  c12 : Outport  Port=14
  c13 : Outport  Port=15
  c14 : Outport  Port=16
  c15 : Outport  Port=17
  wires:
  Concat/1 -> reorder/3(din0)
  Constant3/1 -> reorder/2(en)
  Counter2/1 -> Mux/1
  reorder/1(sync_out) -> Counter2/1, Delay4/1
  reorder/3(dout0) -> Mux/3, Delay1/1
  Concat1/1 -> Mux/2
  Slice6/1 -> Concat1/2
  Slice7/1 -> Concat1/1
  Delay1/1 -> Slice7/1, Slice6/1, Delay5/1
  Mux/1 -> Delay2/1
  Delay5/1 -> Slice20/1, Slice19/1, Slice18/1, Slice17/1, Slice25/1, Slice21/1, Slice9/1, Slice8/1
  Delay4/1 -> sync_out/1
  Slice8/1 -> c0/1
  Slice9/1 -> c1/1
  eq0/1 -> Concat/1
  Slice21/1 -> c2/1
  sync/1 -> reorder/1(sync)
  Slice25/1 -> c3/1
  eq1/1 -> Concat/2
  eq2/1 -> Concat/3
  eq3/1 -> Concat/4
  Delay2/1 -> Slice4/1, Slice3/1, Slice2/1, Slice1/1, Slice27/1, Slice26/1, Slice29/1, Slice28/1
  eq4/1 -> Concat/5
  eq5/1 -> Concat/6
  eq6/1 -> Concat/7
  eq7/1 -> Concat/8
  Slice17/1 -> c4/1
  Slice18/1 -> c5/1
  Slice19/1 -> c6/1
  Slice20/1 -> c7/1
  Slice28/1 -> c8/1
  Slice29/1 -> c9/1
  Slice27/1 -> c11/1
  Slice1/1 -> c12/1
  Slice2/1 -> c13/1
  Slice3/1 -> c14/1
  Slice4/1 -> c15/1
  Slice26/1 -> c10/1

== system rpoco16/seed ==
  BitBasher : xbsIndex_r4/BitBasher  bitexpr=|  display_expr=off  sr_1=1  arith_type1=Unsigned  bin_pt1=0  sr_2=2  arith_type2=Unsigned  bin_pt2=0  sr_3=3  arith_type3=Unsigned  bin_pt3=0  sr_4=4  arith_type4=Unsigned  bin_pt4=0  dbl_ovrd=off  block_type=bitbasher
      | <html><head><meta name="qrichtext" content="1" /><style type="text/css">
      | p, li { white-space: pre-wrap; }
      | </style></head><body style=" font-family:'MS Shell Dlg 2'; font-size:8.25pt; font-weight:400; font-style:normal;">
      | <p style=" margin-top:12px; margin-bottom:12px; margin-left:0px; margin-right:0px; -qt-block-indent:0; text-indent:0px; font-family:'MS Shell Dlg'; font-size:8pt;">seed0={8'h5c, seed[7:0], seed[0:7], 8'ha3}<br />seed1={8'h5c, seed[15:8], seed[8:15], 8'ha3}<br />seed2={8'h5c, seed[23:16], seed[16:23], 8'ha3}<br />seed3={8'h5c, seed[31:24], seed[24:31], 8'ha3}</p></body></html>
      settings: block_version=10.1.3
  Constant : Constant  Value=0
  armed_trigger : casper_library_misc/armed_trigger
  seed_data : Subsystem  Tag=xps:sw_reg  AncestorBlock=xps_library/software register  mask(swreg){mode=one value, io_dir=From Processor, io_delay=0, sample_period=1, names=reg, bitwidths=32, arith_types=0, bin_pts=0, sim_port=on, show_format=off}
      mask prompts: io_dir "I/O direction"; io_delay "I/O delay"; sample_period "Sample period"; names "Name:"; bitwidths "Bitwidth:"; arith_types "Type (ufix=0, fix=1, bool=2):"; bin_pts "Binary pt:"; sim_port "Provide sim input/output?"; show_format "Print format string?"
      mask init:
      | swreg_init(gcb)
      settings: AttributesFormatString=1input
      mask TypeOptions mode: one value | fields of equal size | fields of arbitrary size
      mask Callback mode: swreg_cb(gcb);
      mask TypeOptions io_dir: To Processor | From Processor
      mask Callback io_dir:
      | mask_enables = get_param(gcb, 'MaskEnables');
      | mask_names = get_param(gcb, 'MaskNames');
      | if strcmp(get_param(gcb, 'io_dir'), 'To Processor'),
      |     mask_enables{ismember(mask_names, 'sample_period')} = 'off';
      | else
      |     mask_enables{ismember(mask_names, 'sample_period')} = 'on';
      | end
      | set_param(gcb, 'MaskEnables', mask_enables);
      mask Callback bitwidths: swreg_maskcheck(gcb);
      mask Callback arith_types: [numios, ~, ~, ~, current_types] = swreg_maskcheck(gcb);
      mask Callback bin_pts: swreg_maskcheck(gcb);
  tag scope: seed0=global, seed1=global, seed2=global, seed3=global, seed4=global, seed5=global, seed6=global, seed7=global, seed_ld=global
  wires:
  seed_data/1(in_reg) -> BitBasher/1
  armed_trigger/1 -> [seed_ld]
  [sync_gen] -> armed_trigger/2
  Constant/1 -> seed_data/1(sim_1)
  [arm_rst] -> armed_trigger/1
  BitBasher/1 -> [seed1], [seed0]
  BitBasher/2 -> [seed3], [seed2]
  BitBasher/3 -> [seed5], [seed4]
  BitBasher/4 -> [seed7], [seed6]
